simulink model "open_and_closed_ss_simulink_control101"  (R2025b)
settings: Solver=VariableStepAuto  StartTime=0.0  StopTime=stoptime  RelTol=1e-3
undefined symbols (not defined in the file or in its folder): A, B, C, Kfbk, x0
settings Model: Creator=Anthony Rossiter  LastModifiedBy=Anthony Rossiter

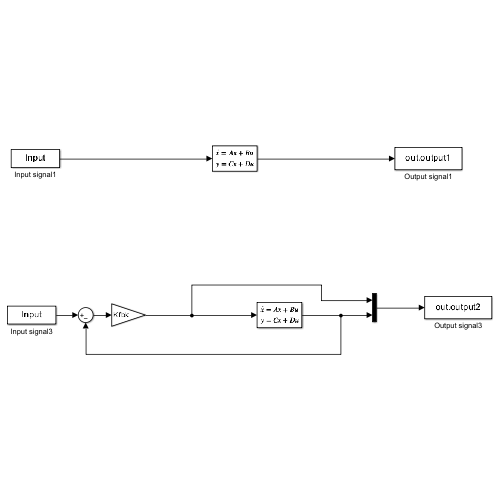
[thumbnail: Simulink's stored preview of the top-level diagram]
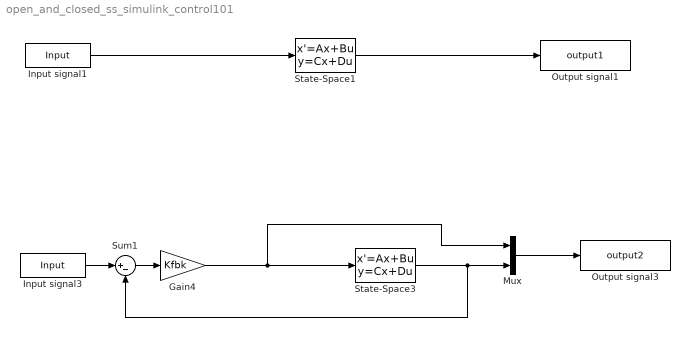
== system open_and_closed_ss_simulink_control101 ==
  Gain4 : Gain  Gain=Kfbk
  Input signal1 : FromWorkspace  VariableName=Input
  Input signal3 : FromWorkspace  VariableName=Input
  Mux : Mux  Inputs=2
  Output signal1 : ToWorkspace  VariableName=output1  SaveFormat=Timeseries  SampleTime=-1
  Output signal3 : ToWorkspace  VariableName=output2  SaveFormat=Timeseries  SampleTime=-1
  State-Space1 : StateSpace  A=A  B=B  C=C  D=0  InitialCondition=x0
  State-Space3 : StateSpace  A=A  B=B  C=C  D=0  InitialCondition=x0
  Sum1 : Sum  Inputs=|+-
  wires:
  State-Space1/1 -> Output signal1/1
  Input signal1/1 -> State-Space1/1
  Input signal3/1 -> Sum1/1
  State-Space3/1 -> Mux/2, Sum1/2
  Sum1/1 -> Gain4/1
  Gain4/1 -> Mux/1, State-Space3/1
  Mux/1 -> Output signal3/1
